simulink model "aaaa"  (R2025a)
settings: Solver=VariableStepAuto  StartTime=0.0  StopTime=12000  FixedStep=1  RelTol=1e-3
settings Model: Creator=user  LastModifiedBy=user

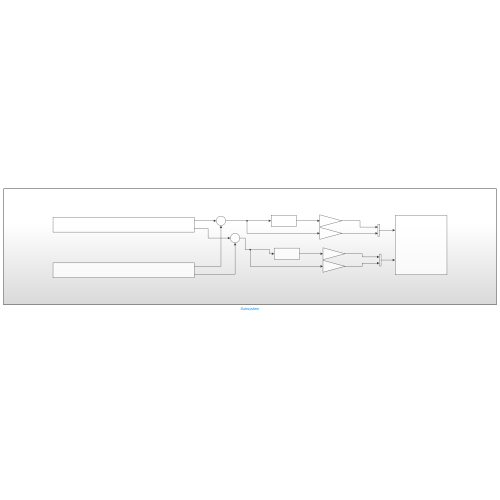
[thumbnail: Simulink's stored preview of the top-level diagram]
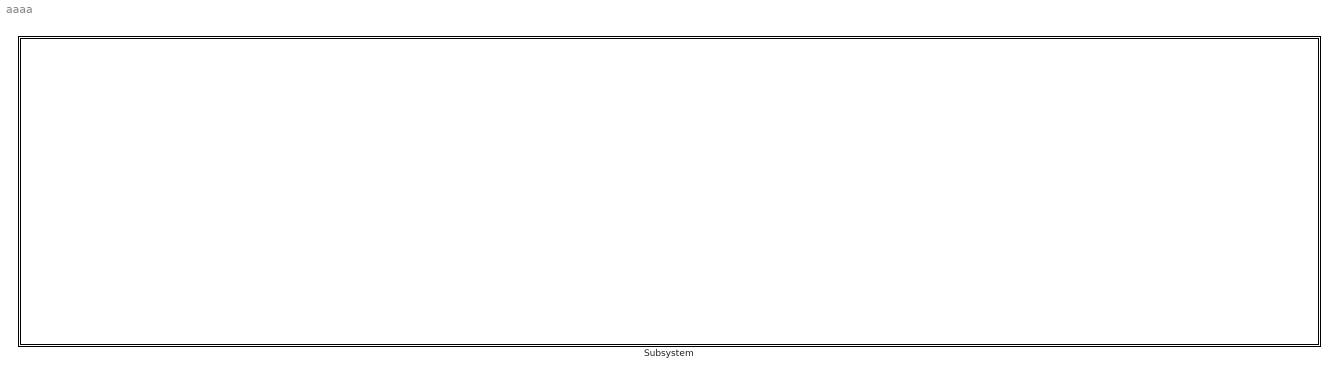
== system aaaa ==
  Subsystem : Subsystem

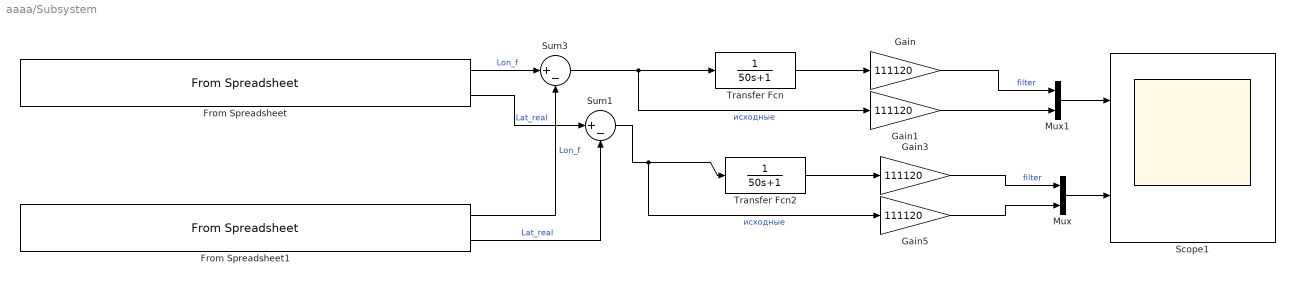
== system aaaa/Subsystem ==
  From Spreadsheet : FromSpreadsheet  FileName=C:\Users\user\Documents\Labworks Romashko\LatLon\LatLon2.xlsx
  From Spreadsheet1 : FromSpreadsheet  FileName=C:\Users\user\Documents\Labworks Romashko\LatLon\LatLon2.xlsx  Range=a2:c2
  Gain{,1,3,5} (4 alike) : Gain  Gain=111120
  Mux : Mux  Inputs=2
  Mux1 : Mux  Inputs=2
  Scope1 : Scope  NumInputPorts=2
      settings: ActiveDisplayYMinimum=-291.41987666104387  ActiveDisplayYMaximum=235.06410590941536
  Sum1 : Sum  Inputs=|+-
  Sum3 : Sum  Inputs=|+-
  Transfer Fcn : TransferFcn  Denominator=[50 1]
  Transfer Fcn2 : TransferFcn  Denominator=[50 1]
  wires:
  Sum3/1 -> Gain1/1, Transfer Fcn/1  "исходные"
  Sum1/1 -> Gain5/1, Transfer Fcn2/1  "исходные"
  Mux1/1 -> Scope1/1
  Gain3/1 -> Mux/1  "filter"
  From Spreadsheet/2 -> Sum1/1  "Lat_real"
  Gain/1 -> Mux1/1  "filter"
  Transfer Fcn/1 -> Gain/1
  Gain5/1 -> Mux/2
  Transfer Fcn2/1 -> Gain3/1
  Gain1/1 -> Mux1/2
  Mux/1 -> Scope1/2
  From Spreadsheet/1 -> Sum3/1  "Lon_f"
  From Spreadsheet1/1 -> Sum3/2  "Lon_f"
  From Spreadsheet1/2 -> Sum1/2  "Lat_real"
